simulink model "PID_Spring_mass_damper"  (R2025b)
settings: Solver=VariableStepAuto  StartTime=0.0  StopTime=30.0  RelTol=1e-3
settings Model: Creator=user  LastModifiedBy=user

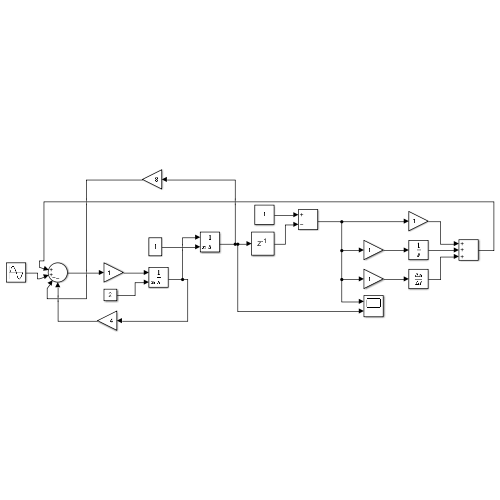
[thumbnail: Simulink's stored preview of the top-level diagram]
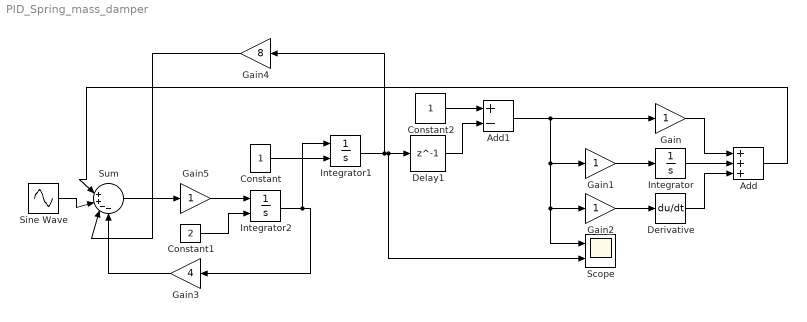
== system PID_Spring_mass_damper ==
  Add : Sum  Inputs=+++
  Add1 : Sum  Inputs=+-
  Constant : Constant
  Constant1 : Constant  Value=2
  Constant2 : Constant
  Delay1 : Delay  DelayLength=1  InputProcessing=Columns as channels (frame based)
  Derivative : Derivative
  Gain{,1..2,5} (4 alike) : Gain
  Gain3 : Gain  Gain=4
  Gain4 : Gain  Gain=8
  Integrator : Integrator
  Integrator1 : Integrator  InitialConditionSource=external  InitialCondition=1
  Integrator2 : Integrator  InitialConditionSource=external  InitialCondition=2
  Scope : Scope  NumInputPorts=2
      settings: ActiveDisplayYMinimum=-0.32509200331759924  ActiveDisplayYMaximum=1.3250920033175995
  Sine Wave : Sin  SampleTime=0
  Sum : Sum  Inputs=||++--
  wires:
  Gain5/1 -> Integrator2/1
  Integrator2/1 -> Gain3/1, Integrator1/1
  Gain4/1 -> Sum/3
  Constant/1 -> Integrator1/2
  Constant1/1 -> Integrator2/2
  Gain3/1 -> Sum/4
  Sum/1 -> Gain5/1
  Integrator1/1 -> Delay1/1, Scope/2, Gain4/1
  Constant2/1 -> Add1/1
  Delay1/1 -> Add1/2
  Add1/1 -> Gain2/1, Scope/1, Gain1/1, Gain/1
  Gain1/1 -> Integrator/1
  Gain2/1 -> Derivative/1
  Gain/1 -> Add/1
  Integrator/1 -> Add/2
  Derivative/1 -> Add/3
  Add/1 -> Sum/1
  Sine Wave/1 -> Sum/2
